simulink model "Copy_of_simuMotor"  (R2014a)
settings: Solver=ode45  StartTime=0.0  StopTime=10.0  MaxStep=0.0001  RelTol=1e-3
values from neighbouring files (symbols this model uses):
  contr = param    [parametres.m]
undefined symbols (not defined in the file or in its folder): param
settings Model: Creator=Etienne  LastModifiedBy=Etienne

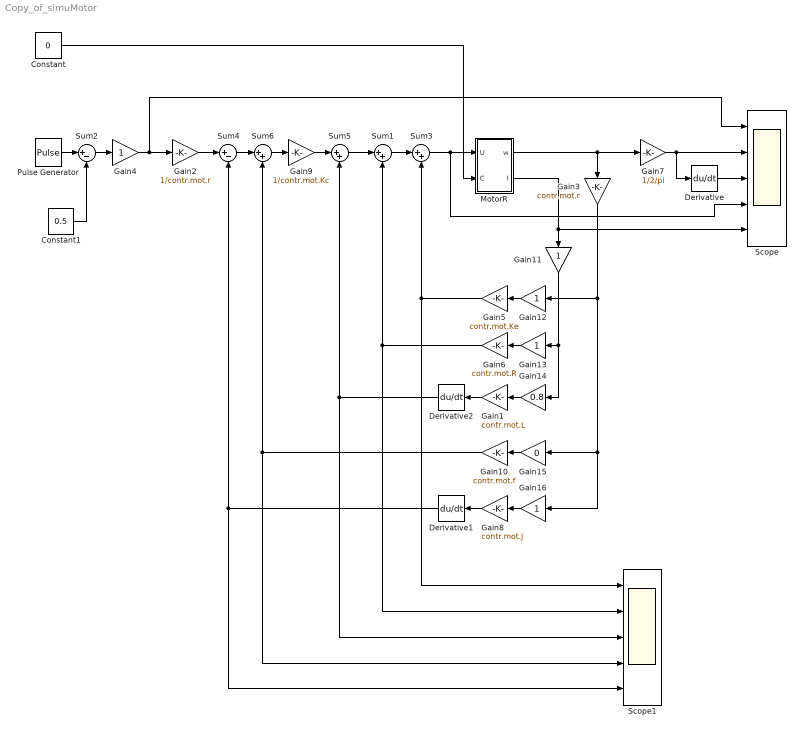
== system Copy_of_simuMotor ==
  Constant : Constant  Value=0
  Constant1 : Constant  Value=0.5
  Derivative : Derivative
  Derivative1 : Derivative
  Derivative2 : Derivative
  Gain1 : Gain  Gain=contr.mot.L
  Gain10 : Gain  Gain=contr.mot.f
  Gain{4,11..13,16} (5 alike) : Gain
  Gain14 : Gain  Gain=0.8
  Gain15 : Gain  Gain=0
  Gain2 : Gain  Gain=1/contr.mot.r
  Gain3 : Gain  Gain=contr.mot.r
  Gain5 : Gain  Gain=contr.mot.Ke
  Gain6 : Gain  Gain=contr.mot.R
  Gain7 : Gain  Gain=1/2/pi
  Gain8 : Gain  Gain=contr.mot.J
  Gain9 : Gain  Gain=1/contr.mot.Kc
  MotorR : Subsystem
  Pulse Generator : DiscretePulseGenerator  PulseType=Time based  Period=1  PulseWidth=50  PhaseDelay=0.25
  Scope : Scope  NumInputPorts=5
      settings: TimeRange=10  YMin=-0.5~-10~-40~-30~-3  YMax=0.5~10~40~30~3  MaxDataPoints=500000
  Scope1 : Scope  NumInputPorts=5
      settings: TimeRange=10  YMin=-30~-5~-1~-1~-0.04  YMax=30~5~1~1~0.04  MaxDataPoints=500000
  Sum{1,3,5..6} (4 alike) : Sum  Inputs=|++
  Sum2 : Sum  Inputs=|+-
  Sum4 : Sum  Inputs=|+-
  wires:
  Constant/1 -> MotorR/2(C)
  Gain5/1 -> Sum3/2, Scope1/1
  MotorR/1(w) -> Gain3/1, Gain7/1
  Gain6/1 -> Scope1/2, Sum1/2
  MotorR/2(I) -> Gain11/1, Scope/5
  Pulse Generator/1 -> Sum2/1
  Sum2/1 -> Gain4/1
  Constant1/1 -> Sum2/2
  Gain4/1 -> Gain2/1, Scope/1
  Gain7/1 -> Derivative/1, Scope/2
  Derivative/1 -> Scope/3
  Gain3/1 -> Gain12/1, Gain15/1, Gain16/1
  Gain8/1 -> Derivative1/1
  Gain2/1 -> Sum4/1
  Sum1/1 -> Sum3/1
  Sum3/1 -> Scope/4, MotorR/1(U)
  Derivative1/1 -> Sum4/2, Scope1/5
  Gain1/1 -> Derivative2/1
  Gain9/1 -> Sum5/1
  Sum5/1 -> Sum1/1
  Derivative2/1 -> Scope1/3, Sum5/2
  Sum6/1 -> Gain9/1
  Sum4/1 -> Sum6/1
  Gain10/1 -> Scope1/4, Sum6/2
  Gain11/1 -> Gain13/1, Gain14/1
  Gain12/1 -> Gain5/1
  Gain13/1 -> Gain6/1
  Gain14/1 -> Gain1/1
  Gain15/1 -> Gain10/1
  Gain16/1 -> Gain8/1

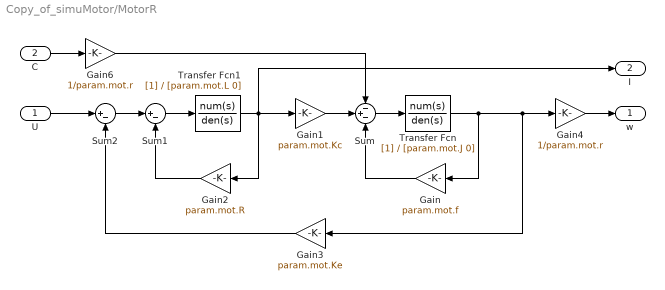
== system Copy_of_simuMotor/MotorR ==
  U : Inport
  C : Inport  Port=2
  Gain : Gain  Gain=param.mot.f
  Gain1 : Gain  Gain=param.mot.Kc
  Gain2 : Gain  Gain=param.mot.R
  Gain3 : Gain  Gain=param.mot.Ke
  Gain4 : Gain  Gain=1/param.mot.r
  Gain6 : Gain  Gain=1/param.mot.r
  Sum : Sum  Inputs=-+-
  Sum1 : Sum  Inputs=|+-
  Sum2 : Sum  Inputs=|+-
  Transfer Fcn : TransferFcn  Denominator=[param.mot.J 0]
  Transfer Fcn1 : TransferFcn  Denominator=[param.mot.L 0]
  w : Outport
  I : Outport  Port=2
  wires:
  Gain1/1 -> Sum/2
  Transfer Fcn/1 -> Gain3/1, Gain4/1, Gain/1
  Gain3/1 -> Sum2/2
  Gain/1 -> Sum/3
  Sum2/1 -> Sum1/1
  Gain2/1 -> Sum1/2
  Sum1/1 -> Transfer Fcn1/1
  U/1 -> Sum2/1
  C/1 -> Gain6/1
  Gain6/1 -> Sum/1
  Gain4/1 -> w/1
  Sum/1 -> Transfer Fcn/1
  Transfer Fcn1/1 -> Gain1/1, I/1, Gain2/1
